simulink model "MMC_Control_PLECS_IFB"  (R2016a)
settings: Solver=VariableStepAuto  SolverMode=SingleTasking  StartTime=0.0  StopTime=0.02  FixedStep=sim_Ts  RelTol=1e-3
undefined symbols (not defined in the file or in its folder): plecs
settings Model: Creator=jason  LastModifiedBy=Francis Chen
settings DebuggingCC: SFUnexpectedBacktrackingDiag=error  SFNoUnconditionalDefaultTransitionDiag=error
settings SFSimCC: SimUseLocalCustomCode=on
settings RTWCC: RTWUseLocalCustomCode=on
settings GRTTargetCC: TargetLangStandard=C99 (ISO)  GeneratePreprocessorConditionals=Use local settings
settings ConfigComp: CovMetricSettings=dwe  CovHtmlReporting=off  CovSaveCumulativeToWorkspaceVar=off  CovSaveSingleToWorkspaceVar=off  CovExternalEMLEnable=on

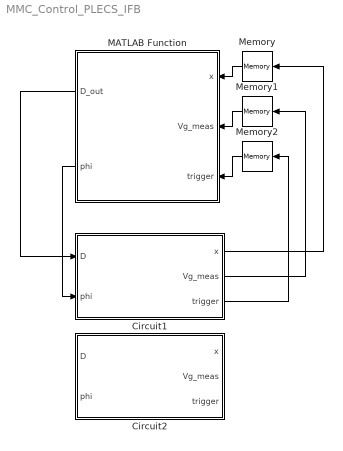
== system MMC_Control_PLECS_IFB ==
  Circuit1 : Subsystem  LoadFcn=plecs('sl', 200);  InitFcn=plecs('sl', 214);  StartFcn=plecs('sl', 208);  StopFcn=plecs('sl', 209);  mask(PlecsCircuit){PLECSData=<binary blob, 32744 chars, not shown>}
      mask prompts: PLECSData "PLECS Data (Do not delete or modify!)"
      mask init:
      | % PLACE CUSTOM INITIALIZATIONS ABOVE
      | % DO NOT REMOVE
      | plecs('sl', 215);
      | % DO NOT REMOVE
      settings: CopyFcn=plecs('sl', 203);  DeleteFcn=plecs('sl', 205);  UndoDeleteFcn=plecs('sl', 206);  PreSaveFcn=plecs('sl', 211);  PostSaveFcn=plecs('sl', 201);  NameChangeFcn=plecs('sl', 210);  DestroyFcn=plecs('sl', 207);  PreCopyFcn=plecs('sl', 216);  OpenFcn=plecs('sl', 202);  ErrorFcn=plerrorfcn
      mask Help: web(['file:///' fullfile(plecsdoc, 'creatingacircuit.html')])
      mask Display: disp('PLECS\nCircuit\nIdeal')
  Circuit2 : Subsystem  LoadFcn=plecs('sl', 200);  InitFcn=plecs('sl', 214);  StartFcn=plecs('sl', 208);  StopFcn=plecs('sl', 209);  mask(PlecsCircuit){PLECSData=<binary blob, 5656 chars, not shown>}
      mask prompts: PLECSData "PLECS Data (Do not delete or modify!)"
      mask init:
      | % PLACE CUSTOM INITIALIZATIONS ABOVE
      | % DO NOT REMOVE
      | plecs('sl', 215);
      | % DO NOT REMOVE
      settings: CopyFcn=plecs('sl', 203);  DeleteFcn=plecs('sl', 205);  UndoDeleteFcn=plecs('sl', 206);  PreSaveFcn=plecs('sl', 211);  PostSaveFcn=plecs('sl', 201);  NameChangeFcn=plecs('sl', 210);  DestroyFcn=plecs('sl', 207);  PreCopyFcn=plecs('sl', 216);  OpenFcn=plecs('sl', 202);  ErrorFcn=plerrorfcn
      mask Help: web(['file:///' fullfile(plecsdoc, 'creatingacircuit.html')])
      mask Display: disp('PLECS\nCircuit\nLeakage')
  MATLAB Function : MATLAB Function  TreatAsAtomicUnit=on
  Memory : Memory  X0=[50,50,50,4,4,4];  InheritSampleTime=on
  Memory1 : Memory  X0=[0,0,0];  InheritSampleTime=on
  Memory2 : Memory  InheritSampleTime=on
  wires:
  Circuit1/3(trigger) -> Memory2/1
  Circuit1/2(Vg_meas) -> Memory1/1
  Circuit1/1(x) -> Memory/1
  MATLAB Function/1(D_out) -> Circuit1/1(D)
  Memory/1 -> MATLAB Function/1(x)
  Memory1/1 -> MATLAB Function/2(Vg_meas)
  Memory2/1 -> MATLAB Function/3(trigger)
  MATLAB Function/2(phi) -> Circuit1/2(phi)

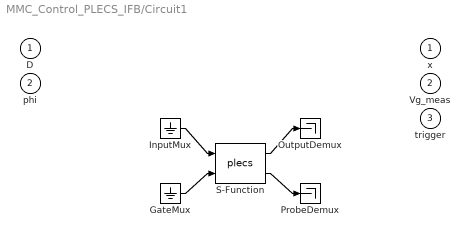
== system MMC_Control_PLECS_IFB/Circuit1 ==
  D : Inport  PortDimensions=6
  phi : Inport  Port=2  PortDimensions=1
  " GateMux " : Ground
  " InputMux " : Ground
  " OutputDemux " : Terminator
  " ProbeDemux " : Terminator
  " S-Function " : S-Function  FunctionName=plecs  SFunctionDeploymentMode=off  EnableBusSupport=off
  x : Outport  PortDimensions=6
  Vg_meas : Outport  Port=2  PortDimensions=3
  trigger : Outport  Port=3  PortDimensions=1
  wires:
  " InputMux "/1 -> " S-Function "/1
  " GateMux "/1 -> " S-Function "/2
  " S-Function "/1 -> " OutputDemux "/1
  " S-Function "/2 -> " ProbeDemux "/1

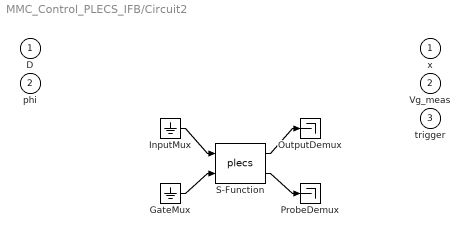
== system MMC_Control_PLECS_IFB/Circuit2 ==
  D : Inport  PortDimensions=6
  phi : Inport  Port=2  PortDimensions=1
  " GateMux " : Ground
  " InputMux " : Ground
  " OutputDemux " : Terminator
  " ProbeDemux " : Terminator
  " S-Function " : S-Function  FunctionName=plecs  SFunctionDeploymentMode=off  EnableBusSupport=off
  x : Outport  PortDimensions=6
  Vg_meas : Outport  Port=2  PortDimensions=3
  trigger : Outport  Port=3  PortDimensions=1
  wires:
  " InputMux "/1 -> " S-Function "/1
  " GateMux "/1 -> " S-Function "/2
  " S-Function "/1 -> " OutputDemux "/1
  " S-Function "/2 -> " ProbeDemux "/1

== matlab function MMC_Control_PLECS_IFB/MATLAB Function ==
  data: x input; D_out output; Vg_meas input; trigger input; nom parameter; phi output
function [D_out,phi]  = MMC_control(x, Vg_meas, trigger,nom)


persistent D_out_val err_int_val phi_val 
if isempty(D_out_val)
    phi_val = 0;
    D_out_val = [0.5; 0.5; 0.5; 0.5; 0.5; 0.5];
    err_int_val = zeros(5,1);
end

if trigger    
Vg_peak = 120; 
Nstate = 6; 
Nout = 5; 

sin_1     = (Vg_meas(1)/Vg_peak);
sin_2     = (Vg_meas(2)/Vg_peak); 
sin_3     = (Vg_meas(3)/Vg_peak); 

phi_1  = asin(sin_1); 
% phi_2  = asin(sin_2); 
% phi_3  = asin(sin_3); 

if (sin_1>=0) && (sin_2>=sin_3)
    phi_1 = pi-phi_1; 
end

if (sin_1<=0) && (sin_2>=sin_3) 
    phi_1 = pi-phi_1; 
end

if phi_1<0 
    phi_1 = phi_1+2*pi;  
end

phi = phi_1; 
tstep   = ceil(interp1(nom.phi,nom.id,phi));
xnom    = nom.x(tstep,:)'; 

% if (abs(sin_3)<0.5)%K13_flag
% K      = nom.K13 (tstep,:,:); 
% yd     = xnom([1:4,6]);
% y      = x([1:4,6]);
% else    
K       = nom.K(tstep,:,:);
yd      = xnom(1:end-1); % last point is not tracked (5 measurements to track)
yd(1:3) = [75;80;85];
y       = x(1:5);
% end

K  = reshape (K,Nstate,Nstate+Nout);
Ki = K       (:,1:Nout); 
Kp = K       (:,Nout+1:end);
tcy     = 1/nom.fsw;
D0      = nom.D (tstep,:)'; %Nominal Duty Cycle

state   =   x - xnom; 
err     =   yd - y; 
err_int =   err*tcy  + err_int_val;


% D-V relationship 1-1, 2-3, 3-1, 4-2, 5-2, 6-3
% Kp(1,2) = 0; Kp(1,3) = 0; 
% Kp(2,1) = 0; Kp(2,2) = 0; 
% Kp(3,2) = 0; Kp(3,3) = 0;
% Kp(4,1) = 0; Kp(4,3) = 0; 
% Kp(5,1) = 0; Kp(5,3) = 0; 
% Kp(6,1) = 0; Kp(6,2) = 0;
% 
% Ki(1,2) = 0; Ki(1,3) = 0; 
% Ki(2,1) = 0; Ki(2,2) = 0; 
% Ki(3,2) = 0; Ki(3,3) = 0;
% Ki(4,1) = 0; Ki(4,3) = 0; 
% Ki(5,1) = 0; Ki(5,3) = 0; 
% Ki(6,1) = 0; Ki(6,2) = 0;



dD      = - Kp*state - Ki*err_int;
D       =   D0+dD;  % pay close attention to the sign!
D       =   max(min(D,0.999),-0.999);

D_out = D;
D_out_val = D;
err_int_val = err_int;
phi_val = phi; 

else
    phi = phi_val; 
    D_out = D_out_val;
end


end %function
